simulink model "windfield_interpolate"  (R2020b)
settings: Solver=VariableStepAuto  StartTime=0.0  StopTime=10.0  RelTol=1e-3
libraries: simulink x1
settings Model: Creator=Dogukan  LastModifiedBy=Dogukan

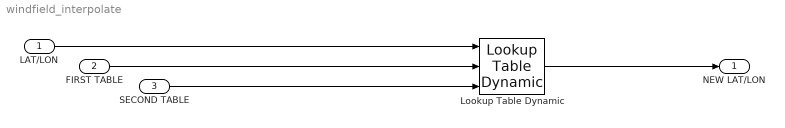
== system windfield_interpolate ==
  LAT/LON : Inport
  FIRST TABLE : Inport  Port=2
  SECOND TABLE : Inport  Port=3
  Lookup Table Dynamic : simulink/Lookup Tables/Lookup Table Dynamic  LookUpMeth=Interpolation-Use End Values  OutDataType=fixdt('double')  OutScaling=2^-10  OutputDataTypeScalingMode=Specify via dialog  OutDataTypeStr=double  DoSatur=off
  NEW LAT/LON : Outport
  wires:
  FIRST TABLE/1 -> Lookup Table Dynamic/2
  SECOND TABLE/1 -> Lookup Table Dynamic/3
  LAT/LON/1 -> Lookup Table Dynamic/1
  Lookup Table Dynamic/1 -> NEW LAT/LON/1
